simulink model "flightControlSystem"  (R2023a)
settings: Solver=ode3  StartTime=0  StopTime=inf  FixedStep=Ts  RelTol=1e-3  EnableMultiTasking=on
undefined symbols (not defined in the file): codertarget, Controller, DiscIntNeverNeededParam, Discrete, Estimator, g, init, Sensors, Time, Ts, var_acc_angle_N, var_bias_gyr_N, var_gyro_p_N, Vehicle
libraries: simulink x37, slpidlib x4, ctrlSharedLib x4, sharedtransform x3, parrotlib x1
(part 3 of 3)

== matlab function flightControlSystem/Control System/Path Planning/Tracking ==
  data: Trck_ena input; u input; x_inc output; y_inc output
function [x_inc, y_inc] = XY_Ctrl(Trck_ena,u)
%%%% Tuning parameters
Gain_x_dir = 0.001;
Gain_y_dir = 0.001;
%%
if Trck_ena ==  1
    x_inc = u(1)*Gain_x_dir;
    y_inc = u(2)*Gain_y_dir;
else
    x_inc = 0;
    y_inc = 0;
end
end

== matlab function flightControlSystem/Control System/Path Planning/Slow Movement  ==
  data: Trig_End input; x_inc_F output; U_prev input; Circle_Detected input; Land_End input; y_inc_F output
function [x_inc_F, y_inc_F] = XY_Ctrl(Trig_End,U_prev,Circle_Detected,Land_End)
%%%% Tuning parameters
Gain_x_dir = 0.0005;
Gain_y_dir = 0.0005;
%%
if (Trig_End == 0) && (Circle_Detected == 0) && (Land_End == 0)
    x_inc_F = U_prev(1)*Gain_x_dir;
    y_inc_F = U_prev(2)*Gain_y_dir;
else
    x_inc_F = 0;
    y_inc_F = 0;
end
end
